simulink model "pendule_inverse"  (R2023b)
settings: Solver=ode45  StartTime=0.0  StopTime=5  RelTol=1e-3
values from neighbouring files (symbols this model uses):
  K = [30 10 10 10]    [init.m]    (also in matrices.m = -place(A,B,V))
  ue = 0    [init.m]    (also in matrices.m)
  x0 = [0 pi/5 0 0]'    [init.m]    (also in matrices.m = [0 ,pi/20 ,0 , 0])
  xe = [0 0 0 0]'    [init.m]    (also in matrices.m = [0, 0, 0, 0])
undefined symbols (not defined in the file or in its folder): DiscIntNeverNeededParam
libraries: simulink x1
settings Model: Creator=fhudrisi  LastModifiedBy=lae
settings OptimizationCC: ReuseModelBlockBuffer=off
settings DebuggingCC: AlgebraicLoopMsg=none  UnconnectedInputMsg=warning  UnconnectedOutputMsg=warning  UnconnectedLineMsg=warning
settings ModelReferenceCC: EnableRefExpFcnMdlSchedulingChecks=on
settings RTWCC: DLArmComputeVersion=19.05

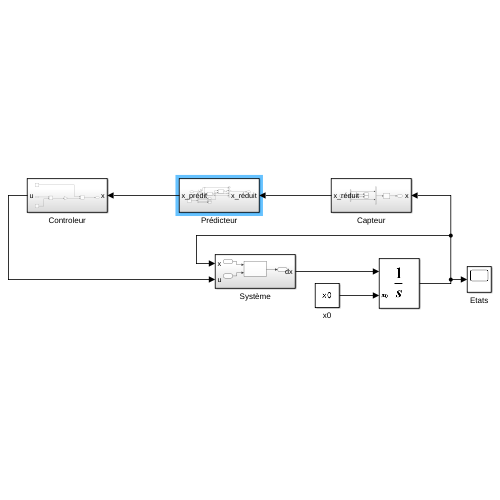
[thumbnail: Simulink's stored preview of the top-level diagram]
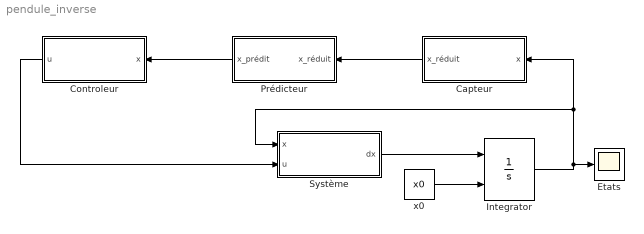
== system pendule_inverse ==
  Capteur : Subsystem
  Controleur : Subsystem
  Etats : Scope
  Integrator : Integrator  InitialConditionSource=external
  Prédicteur : Subsystem
  Système : Subsystem
  x0 : Constant  Value=x0
  wires:
  Système/1(dx) -> Integrator/1
  x0/1 -> Integrator/2
  Integrator/1 -> Système/1(x), Capteur/1(x), Etats/1
  Controleur/1(u) -> Système/2(u)
  Capteur/1(x_réduit) -> Prédicteur/1(x_réduit)
  Prédicteur/1(x_prédit) -> Controleur/1(x)

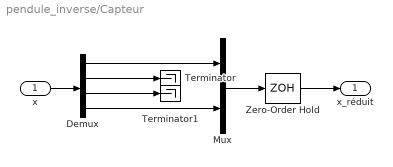
== system pendule_inverse/Capteur ==
  x : Inport
  Demux : Demux
  Mux : Mux  Inputs=2
  Terminator : Terminator
  Terminator1 : Terminator
  Zero-Order Hold : ZeroOrderHold  SampleTime=-1
  x_réduit : Outport
  wires:
  x/1 -> Demux/1
  Demux/1 -> Mux/1
  Demux/4 -> Mux/2
  Demux/2 -> Terminator/1
  Demux/3 -> Terminator1/1
  Mux/1 -> Zero-Order Hold/1
  Zero-Order Hold/1 -> x_réduit/1

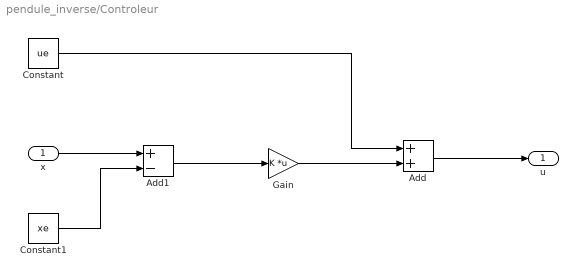
== system pendule_inverse/Controleur ==
  x : Inport  PortDimensions=4
  Add : Sum
  Add1 : Sum  Inputs=+-
  Constant : Constant  Value=ue
  Constant1 : Constant  Value=xe
  Gain : Gain  Gain=K  Multiplication=Matrix(K*u)
  u : Outport
  wires:
  x/1 -> Add1/1
  Constant1/1 -> Add1/2
  Add1/1 -> Gain/1
  Constant/1 -> Add/1
  Gain/1 -> Add/2
  Add/1 -> u/1

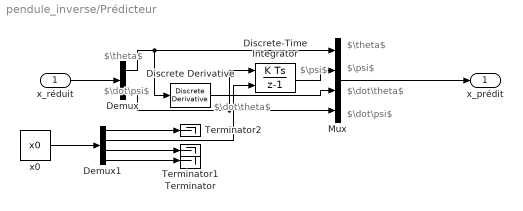
== system pendule_inverse/Prédicteur ==
  note: $\theta$
  note: $\dot\psi$
  note: $\dot\theta$
  note: $\psi$
  note: $\dot\psi$
  note: $\theta$
  note: $\psi$
  note: $\dot\theta$
  x_réduit : Inport  PortDimensions=2
  Demux : Demux  Outputs=2
  Demux1 : Demux
  Discrete Derivative : simulink/Discrete/Discrete Derivative  gainval=1.0  ICPrevScaledInput=0.0  OutMin=[]  OutMax=[]  OutDataType=fixdt(1, 16)  OutScaling=2^-10  DoSatur=off
  Discrete-Time Integrator : DiscreteIntegrator  InitialConditionSource=external  SampleTime=0.005  ICPrevOutput=DiscIntNeverNeededParam  ICPrevScaledInput=DiscIntNeverNeededParam
  Mux : Mux
  Terminator : Terminator
  Terminator1 : Terminator
  Terminator2 : Terminator
  x0 : Constant  Value=x0
  x_prédit : Outport  PortDimensions=4
  wires:
  Mux/1 -> x_prédit/1
  x_réduit/1 -> Demux/1
  Demux/1 -> Discrete Derivative/1, Mux/1
  Demux/2 -> Mux/4, Discrete-Time Integrator/1
  x0/1 -> Demux1/1
  Demux1/1 -> Terminator2/1
  Demux1/3 -> Terminator1/1
  Demux1/4 -> Terminator/1
  Discrete-Time Integrator/1 -> Mux/2
  Discrete Derivative/1 -> Mux/3
  Demux1/2 -> Discrete-Time Integrator/2

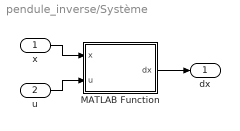
== system pendule_inverse/Système ==
  x : Inport
  u : Inport  Port=2
  MATLAB Function : MATLAB Function  TreatAsAtomicUnit=on
  dx : Outport
  wires:
  MATLAB Function/1(dx) -> dx/1
  x/1 -> MATLAB Function/1(x)
  u/1 -> MATLAB Function/2(u)

== matlab function pendule_inverse/Système/MATLAB Function ==
  data: x input; u input; dx output
function dx   = fonction( x, u)
%   Dynamic equations of motion of the segway on an axis.
%   Inputs: - x = [theta psi dtheta dpsi]
%               theta: average angle of the wheels      [rad]
%               psi: body pitch angle                   [rad]
%               dtheta: average velocity of the wheels  [rad/s]
%               dpsi: body pitch velocity               [rad/s]
%          - u: DC motor voltage (same value for both motors) [V]

    % State
    psi = x(2);
    dtheta = x(3);
    dpsi = x(4);

    % Parameters
    
    g = 9.81;           % gravity acceleration [m/sec^2]
    m = 0.03;           % wheel weight [kg]
    R = 0.04;           % wheel radius [m]
    Jw = m*R^2/2;       % wheel inertia moment [kg*m^2]
    M = 0.6;            % body weight [kg]
    H = 0.144;          % body height [m]
    L = H/2;            % distance of the center of mass from the wheel axle [m]
    Jpsi = M*L^2/3;     % body pitch inertia [kgm^2]
    Jm = 1e-5;          % DC motor inertia moment [kgm^2]
    Rm = 6.69;          % DC motor resistance [Ohm]
    Kb = 0.468;         % DC motor back EMF constant [Vsec/rad]
    Kt = 0.317;         % DC motor torque constant [Nm/A]
    n = 1;              % gear ratio
    fm = 0.0022;        % friction coefficient between body and DC motor
    fw = 0;             % friction coefficient between wheel and floor
    
    % Equations of motion
    c1 = (2*m+M)*R^2 + 2*Jw + 2*n^2*Jm;
    c2 = M*L*R*cos(psi) - 2*n^2*Jm;
    c3 = -M*L*R*dpsi^2*sin(psi);
    c4 = M*L^2 + Jpsi + 2*n^2*Jm;
    c5 = -M*g*L*sin(psi);

    alpha = Kt/Rm;
    beta = Kt*Kb/Rm + fm;

    Ftheta = alpha*(2*u) - 2*(beta+fw)*dtheta + 2*beta*dpsi;
    Fpsi = -alpha*(2*u) + 2*beta*dtheta - 2*beta*dpsi;

    ddtheta = (c4*c3 - c2*c5 + c4*Ftheta - c2*Fpsi)/(c4*c1 - c2^2);
    ddpsi = (Fpsi- c2*ddtheta - c5)/c4;
    dx = [dtheta dpsi ddtheta ddpsi]';

end
